simulink model "resolved_acceleration_controller"  (R2016a)
settings: Solver=VariableStepAuto  StartTime=0.0  StopTime=10.0  RelTol=1e-3
InitFcn:
  | % Parametros
  | m = 1.83;
  | L = 0.09;
  | r = 0.072;
  | Jw = 8.1e-4;
  | J = 2.125;
  | 
  | a1 =  2*r^2*m/(2*r^2*m+3*Jw); % não está sendo utilizado (foi parte do cálculo de outras constantes)
  | a2 = 3*Jw/(2*r^2*m+3*Jw);
  | b1 = r/(2*r^2*m+3*Jw);
  | b2 = r*L/(J*r^2+3*Jw*L^2);
values from neighbouring files (symbols this model uses):
  Kix = 25    [resultados_velocidade_linear_constante.mat]
  Kiy = 25    [resultados_velocidade_linear_constante.mat]
  Kpphi = 2.25    [resultados_velocidade_linear_constante.mat]
  Kpx = 10    [resultados_velocidade_linear_constante.mat]
  Kpy = 10    [resultados_velocidade_linear_constante.mat]
  Kvphi = 3    [resultados_velocidade_linear_constante.mat]
settings Model: Creator=Pichau  LastModifiedBy=Pichau

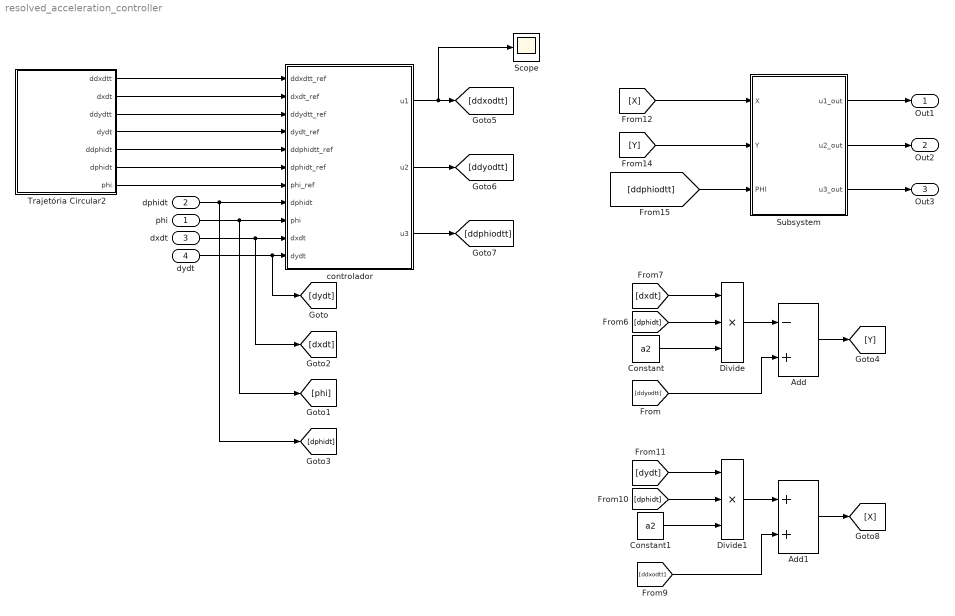
== system resolved_acceleration_controller ==
  phi : Inport
  dphidt : Inport  Port=2
  dxdt : Inport  Port=3
  dydt : Inport  Port=4
  Add : Sum  Inputs=-+
  Add1 : Sum
  Constant : Constant  Value=a2
  Constant1 : Constant  Value=a2
  Divide : Product  Inputs=***
  Divide1 : Product  Inputs=***
  Scope : Scope
  Subsystem : Subsystem
  Trajetória Circular2 : Subsystem
  controlador : Subsystem
  Out1 : Outport
  Out2 : Outport  Port=2
  Out3 : Outport  Port=3
  wires:
  controlador/1(u1) -> Scope/1, [ddxodtt]
  controlador/2(u2) -> [ddyodtt]
  controlador/3(u3) -> [ddphiodtt]
  phi/1 -> [phi], controlador/9(phi)
  dphidt/1 -> [dphidt], controlador/8(dphidt)
  dxdt/1 -> [dxdt], controlador/10(dxdt)
  dydt/1 -> [dydt], controlador/11(dydt)
  Constant/1 -> Divide/3
  [dphidt] -> Divide/2
  [dxdt] -> Divide/1
  Divide/1 -> Add/1
  [ddyodtt] -> Add/2
  Add/1 -> [Y]
  Constant1/1 -> Divide1/3
  [dphidt] -> Divide1/2
  [dydt] -> Divide1/1
  Divide1/1 -> Add1/1
  [ddxodtt] -> Add1/2
  Add1/1 -> [X]
  [X] -> Subsystem/1(X)
  [Y] -> Subsystem/2(Y)
  [ddphiodtt] -> Subsystem/3(PHI)
  Subsystem/1(u1_out) -> Out1/1
  Subsystem/2(u2_out) -> Out2/1
  Subsystem/3(u3_out) -> Out3/1
  Trajetória Circular2/1(ddxdtt) -> controlador/1(ddxdtt_ref)
  Trajetória Circular2/2(dxdt) -> controlador/2(dxdt_ref)
  Trajetória Circular2/3(ddydtt) -> controlador/3(ddydtt_ref)
  Trajetória Circular2/4(dydt) -> controlador/4(dydt_ref)
  Trajetória Circular2/5(ddphidt) -> controlador/5(ddphidtt_ref)
  Trajetória Circular2/6(dphidt) -> controlador/6(dphidt_ref)
  Trajetória Circular2/7(phi) -> controlador/7(phi_ref)

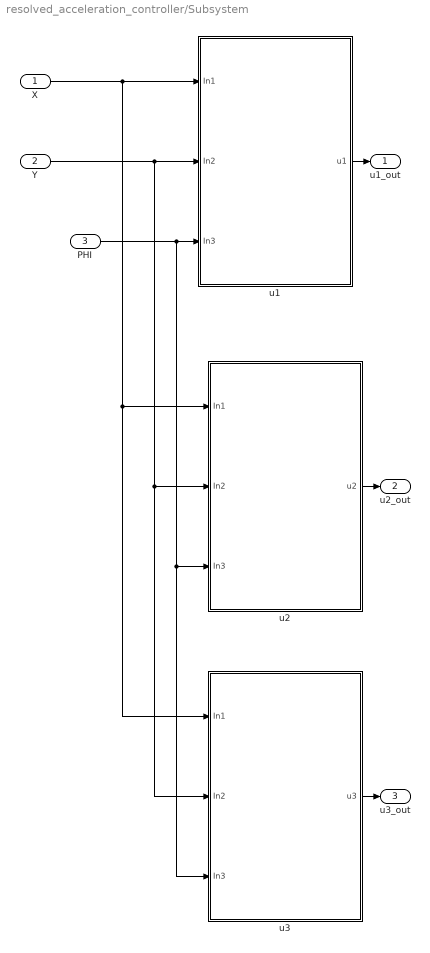
== system resolved_acceleration_controller/Subsystem ==
  X : Inport
  Y : Inport  Port=2
  PHI : Inport  Port=3
  u1 : Subsystem
  u2 : Subsystem
  u3 : Subsystem
  u1_out : Outport
  u2_out : Outport  Port=2
  u3_out : Outport  Port=3
  wires:
  Y/1 -> u3/2(In2), u2/2(In2), u1/2(In2)
  PHI/1 -> u3/3(In3), u2/3(In3), u1/3(In3)
  X/1 -> u3/1(In1), u2/1(In1), u1/1(In1)
  u1/1(u1) -> u1_out/1
  u3/1(u3) -> u3_out/1
  u2/1(u2) -> u2_out/1

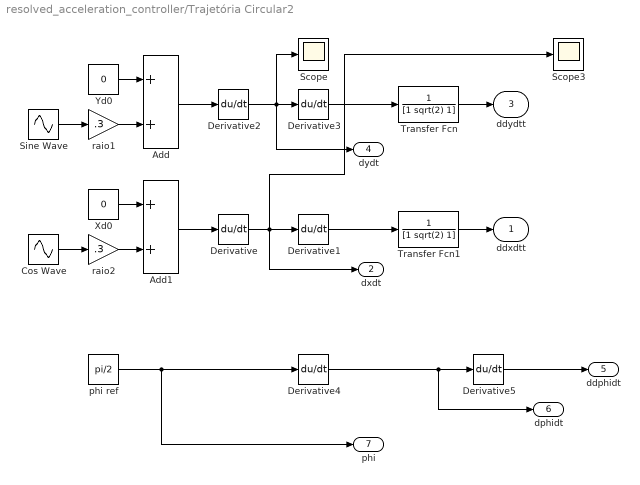
== system resolved_acceleration_controller/Trajetória Circular2 ==
  Add : Sum
  Add1 : Sum
  Cos Wave : Sin  Frequency=0.3  Phase=pi/2  SampleTime=0
  Derivative{,1..5} (6 alike) : Derivative
  Scope : Scope
  Scope3 : Scope
  Sine Wave : Sin  Frequency=0.3  SampleTime=0
  Transfer Fcn : TransferFcn  Denominator=[1 sqrt(2) 1]
  Transfer Fcn1 : TransferFcn  Denominator=[1 sqrt(2) 1]
  Xd0 : Constant  Value=0
  Yd0 : Constant  Value=0
  phi ref : Constant  Value=pi/2
  raio1 : Gain  Gain=.3
  raio2 : Gain  Gain=.3
  ddxdtt : Outport
  dxdt : Outport  Port=2
  ddydtt : Outport  Port=3
  dydt : Outport  Port=4
  ddphidt : Outport  Port=5
  dphidt : Outport  Port=6
  phi : Outport  Port=7
  wires:
  Transfer Fcn1/1 -> ddxdtt/1
  Transfer Fcn/1 -> ddydtt/1
  Derivative5/1 -> ddphidt/1
  Derivative1/1 -> Transfer Fcn1/1
  Derivative3/1 -> Transfer Fcn/1
  Derivative2/1 -> Derivative3/1, Scope/1, dydt/1
  Derivative/1 -> Scope3/1, Derivative1/1, dxdt/1
  Sine Wave/1 -> raio1/1
  raio1/1 -> Add/2
  Add/1 -> Derivative2/1
  Add1/1 -> Derivative/1
  raio2/1 -> Add1/2
  Cos Wave/1 -> raio2/1
  Xd0/1 -> Add1/1
  Yd0/1 -> Add/1
  phi ref/1 -> Derivative4/1, phi/1
  Derivative4/1 -> Derivative5/1, dphidt/1

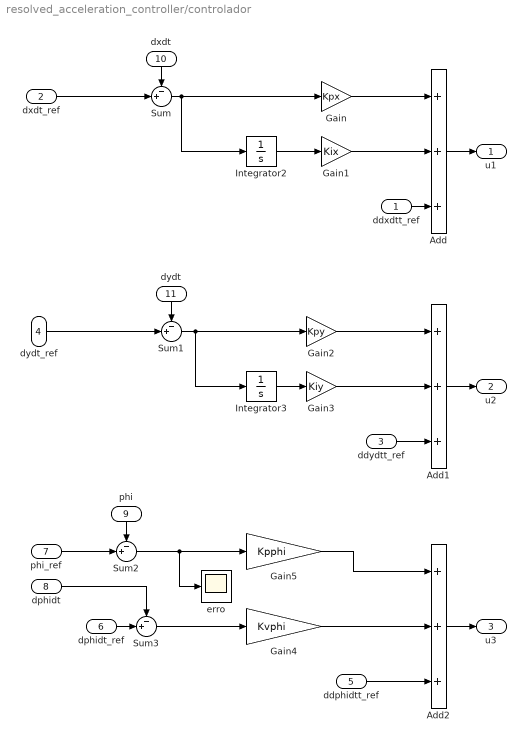
== system resolved_acceleration_controller/controlador ==
  ddxdtt_ref : Inport
  dxdt_ref : Inport  Port=2
  ddydtt_ref : Inport  Port=3
  dydt_ref : Inport  Port=4
  ddphidtt_ref : Inport  Port=5
  dphidt_ref : Inport  Port=6
  phi_ref : Inport  Port=7
  dphidt : Inport  Port=8
  phi : Inport  Port=9
  dxdt : Inport  Port=10
  dydt : Inport  Port=11
  Add : Sum  Inputs=+++
  Add1 : Sum  Inputs=+++
  Add2 : Sum  Inputs=+++
  Gain : Gain  Gain=Kpx
  Gain1 : Gain  Gain=Kix
  Gain2 : Gain  Gain=Kpy
  Gain3 : Gain  Gain=Kiy
  Gain4 : Gain  Gain=Kvphi
  Gain5 : Gain  Gain=Kpphi
  Integrator2 : Integrator
  Integrator3 : Integrator
  Sum{,1..3} (4 alike) : Sum  Inputs=-+|
  erro : Scope
  u1 : Outport
  u2 : Outport  Port=2
  u3 : Outport  Port=3
  wires:
  Sum2/1 -> Gain5/1, erro/1
  Sum1/1 -> Gain2/1, Integrator3/1
  Gain1/1 -> Add/2
  Integrator2/1 -> Gain1/1
  dydt_ref/1 -> Sum1/2
  Add/1 -> u1/1
  Gain2/1 -> Add1/1
  Integrator3/1 -> Gain3/1
  dphidt/1 -> Sum3/1
  Gain4/1 -> Add2/2
  Sum/1 -> Gain/1, Integrator2/1
  Gain3/1 -> Add1/2
  Gain5/1 -> Add2/1
  Sum3/1 -> Gain4/1
  ddphidtt_ref/1 -> Add2/3
  ddydtt_ref/1 -> Add1/3
  Add1/1 -> u2/1
  ddxdtt_ref/1 -> Add/3
  phi/1 -> Sum2/1
  Add2/1 -> u3/1
  dxdt_ref/1 -> Sum/2
  dxdt/1 -> Sum/1
  phi_ref/1 -> Sum2/2
  Gain/1 -> Add/1
  dydt/1 -> Sum1/1
  dphidt_ref/1 -> Sum3/2

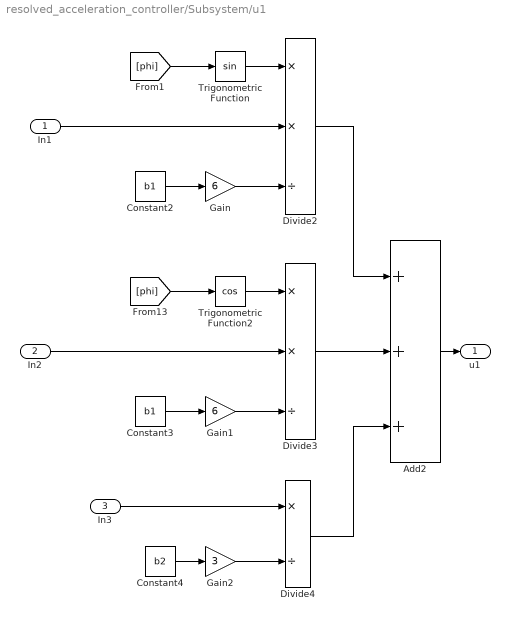
== system resolved_acceleration_controller/Subsystem/u1 ==
  In1 : Inport
  In2 : Inport  Port=2
  In3 : Inport  Port=3
  Add2 : Sum  Inputs=+++
  Constant2 : Constant  Value=b1
  Constant3 : Constant  Value=b1
  Constant4 : Constant  Value=b2
  Divide2 : Product  Inputs=**/
  Divide3 : Product  Inputs=**/
  Divide4 : Product  Inputs=*/
  Gain : Gain  Gain=6
  Gain1 : Gain  Gain=6
  Gain2 : Gain  Gain=3
  Trigonometric Function : Trigonometry
  Trigonometric Function2 : Trigonometry  Operator=cos
  u1 : Outport
  wires:
  Add2/1 -> u1/1
  Divide3/1 -> Add2/2
  Divide4/1 -> Add2/3
  In1/1 -> Divide2/2
  Gain2/1 -> Divide4/2
  Constant2/1 -> Gain/1
  Gain/1 -> Divide2/3
  [phi] -> Trigonometric Function/1
  Divide2/1 -> Add2/1
  Constant4/1 -> Gain2/1
  [phi] -> Trigonometric Function2/1
  Trigonometric Function2/1 -> Divide3/1
  In2/1 -> Divide3/2
  Constant3/1 -> Gain1/1
  Gain1/1 -> Divide3/3
  Trigonometric Function/1 -> Divide2/1
  In3/1 -> Divide4/1

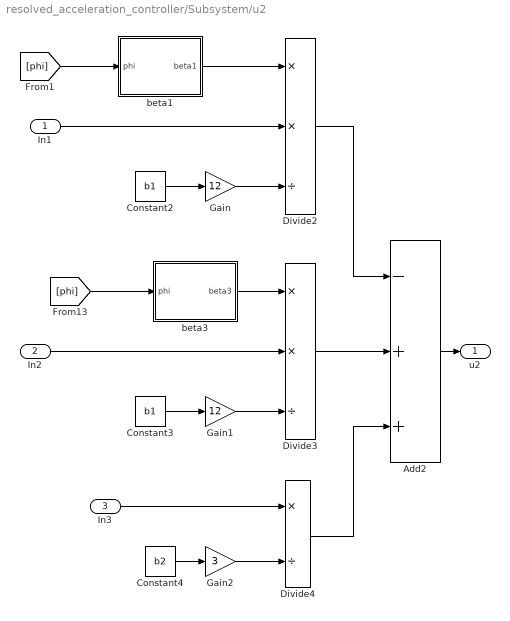
== system resolved_acceleration_controller/Subsystem/u2 ==
  In1 : Inport
  In2 : Inport  Port=2
  In3 : Inport  Port=3
  Add2 : Sum  Inputs=-++
  Constant2 : Constant  Value=b1
  Constant3 : Constant  Value=b1
  Constant4 : Constant  Value=b2
  Divide2 : Product  Inputs=**/
  Divide3 : Product  Inputs=**/
  Divide4 : Product  Inputs=*/
  Gain : Gain  Gain=12
  Gain1 : Gain  Gain=12
  Gain2 : Gain  Gain=3
  beta1 : Subsystem
  beta3 : Subsystem
  u2 : Outport
  wires:
  In3/1 -> Divide4/1
  beta1/1(beta1) -> Divide2/1
  Gain1/1 -> Divide3/3
  Constant3/1 -> Gain1/1
  In2/1 -> Divide3/2
  beta3/1(beta3) -> Divide3/1
  [phi] -> beta3/1(phi)
  Constant4/1 -> Gain2/1
  Divide2/1 -> Add2/1
  [phi] -> beta1/1(phi)
  Gain/1 -> Divide2/3
  Constant2/1 -> Gain/1
  Gain2/1 -> Divide4/2
  In1/1 -> Divide2/2
  Divide4/1 -> Add2/3
  Divide3/1 -> Add2/2
  Add2/1 -> u2/1

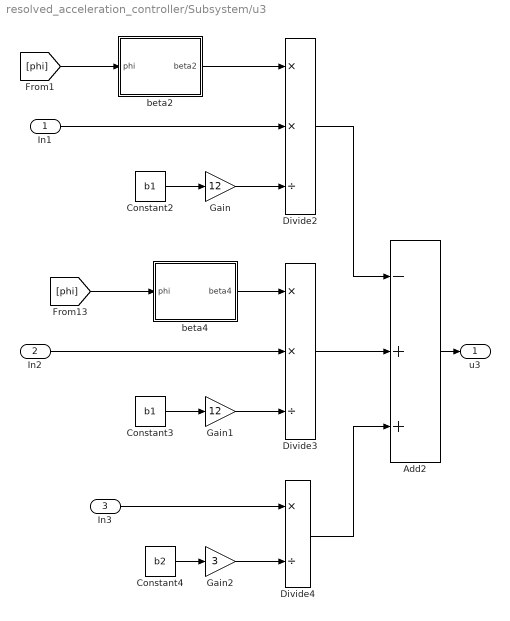
== system resolved_acceleration_controller/Subsystem/u3 ==
  In1 : Inport
  In2 : Inport  Port=2
  In3 : Inport  Port=3
  Add2 : Sum  Inputs=-++
  Constant2 : Constant  Value=b1
  Constant3 : Constant  Value=b1
  Constant4 : Constant  Value=b2
  Divide2 : Product  Inputs=**/
  Divide3 : Product  Inputs=**/
  Divide4 : Product  Inputs=*/
  Gain : Gain  Gain=12
  Gain1 : Gain  Gain=12
  Gain2 : Gain  Gain=3
  beta2 : Subsystem
  beta4 : Subsystem
  u3 : Outport
  wires:
  In3/1 -> Divide4/1
  beta2/1(beta2) -> Divide2/1
  Gain1/1 -> Divide3/3
  Constant3/1 -> Gain1/1
  In2/1 -> Divide3/2
  beta4/1(beta4) -> Divide3/1
  [phi] -> beta4/1(phi)
  Constant4/1 -> Gain2/1
  Divide2/1 -> Add2/1
  [phi] -> beta2/1(phi)
  Gain/1 -> Divide2/3
  Constant2/1 -> Gain/1
  Gain2/1 -> Divide4/2
  In1/1 -> Divide2/2
  Divide4/1 -> Add2/3
  Divide3/1 -> Add2/2
  Add2/1 -> u3/1

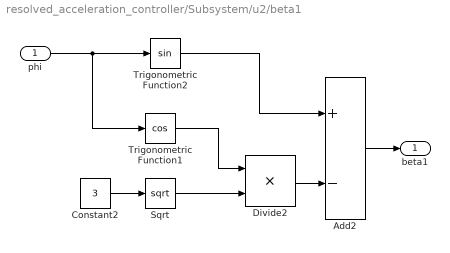
== system resolved_acceleration_controller/Subsystem/u2/beta1 ==
  phi : Inport
  Add2 : Sum  Inputs=+-
  Constant2 : Constant  Value=3
  Divide2 : Product  Inputs=**
  Sqrt : Sqrt  SaturateOnIntegerOverflow=on
  Trigonometric Function1 : Trigonometry  Operator=cos
  Trigonometric Function2 : Trigonometry
  beta1 : Outport
  wires:
  Trigonometric Function2/1 -> Add2/1
  phi/1 -> Trigonometric Function1/1, Trigonometric Function2/1
  Constant2/1 -> Sqrt/1
  Sqrt/1 -> Divide2/2
  Add2/1 -> beta1/1
  Trigonometric Function1/1 -> Divide2/1
  Divide2/1 -> Add2/2

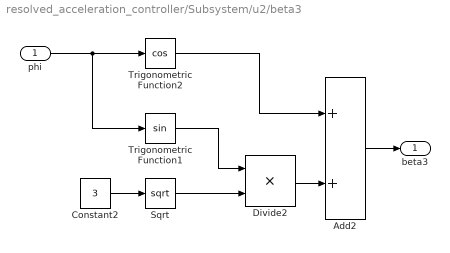
== system resolved_acceleration_controller/Subsystem/u2/beta3 ==
  phi : Inport
  Add2 : Sum
  Constant2 : Constant  Value=3
  Divide2 : Product  Inputs=**
  Sqrt : Sqrt  SaturateOnIntegerOverflow=on
  Trigonometric Function1 : Trigonometry
  Trigonometric Function2 : Trigonometry  Operator=cos
  beta3 : Outport
  wires:
  Trigonometric Function2/1 -> Add2/1
  phi/1 -> Trigonometric Function1/1, Trigonometric Function2/1
  Constant2/1 -> Sqrt/1
  Sqrt/1 -> Divide2/2
  Add2/1 -> beta3/1
  Trigonometric Function1/1 -> Divide2/1
  Divide2/1 -> Add2/2

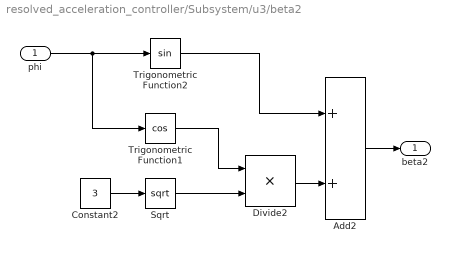
== system resolved_acceleration_controller/Subsystem/u3/beta2 ==
  phi : Inport
  Add2 : Sum
  Constant2 : Constant  Value=3
  Divide2 : Product  Inputs=**
  Sqrt : Sqrt  SaturateOnIntegerOverflow=on
  Trigonometric Function1 : Trigonometry  Operator=cos
  Trigonometric Function2 : Trigonometry
  beta2 : Outport
  wires:
  Divide2/1 -> Add2/2
  Trigonometric Function1/1 -> Divide2/1
  Add2/1 -> beta2/1
  Sqrt/1 -> Divide2/2
  Constant2/1 -> Sqrt/1
  phi/1 -> Trigonometric Function2/1, Trigonometric Function1/1
  Trigonometric Function2/1 -> Add2/1

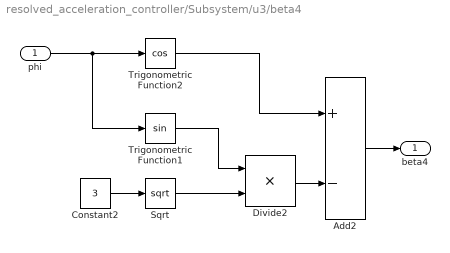
== system resolved_acceleration_controller/Subsystem/u3/beta4 ==
  phi : Inport
  Add2 : Sum  Inputs=+-
  Constant2 : Constant  Value=3
  Divide2 : Product  Inputs=**
  Sqrt : Sqrt  SaturateOnIntegerOverflow=on
  Trigonometric Function1 : Trigonometry
  Trigonometric Function2 : Trigonometry  Operator=cos
  beta4 : Outport
  wires:
  Divide2/1 -> Add2/2
  Trigonometric Function1/1 -> Divide2/1
  Add2/1 -> beta4/1
  Sqrt/1 -> Divide2/2
  Constant2/1 -> Sqrt/1
  phi/1 -> Trigonometric Function2/1, Trigonometric Function1/1
  Trigonometric Function2/1 -> Add2/1
